simulink model "groudstation20180903"  (R2017b)
settings: Solver=VariableStepAuto  StartTime=0.0  StopTime=inf  RelTol=1e-3
undefined symbols (not defined in the file or in its folder): serial
libraries: instrumentlib x2
settings Model: Creator=E6320  LastModifiedBy=E6320

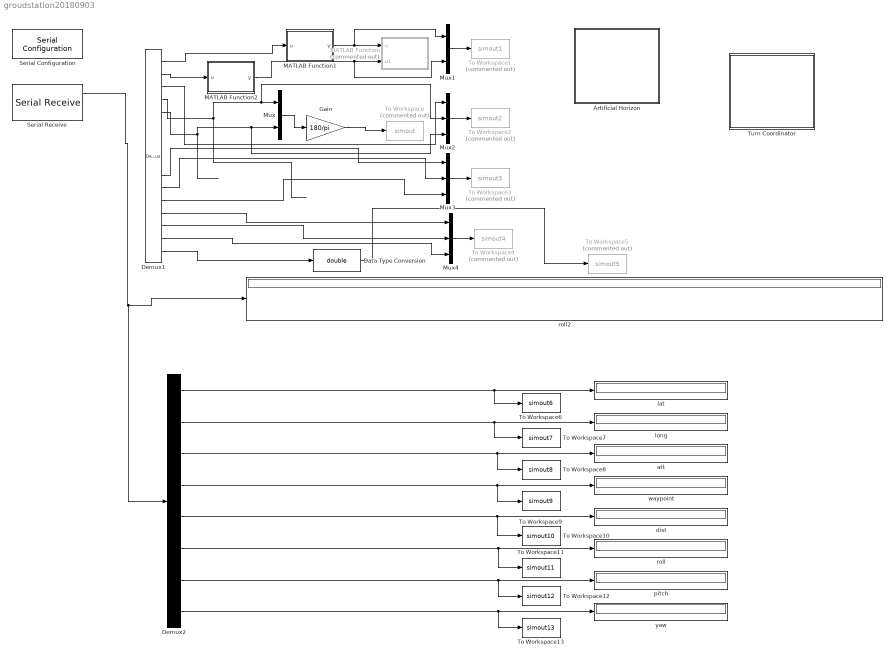
== system groudstation20180903 ==
  Artificial Horizon : Subsystem  DialogController=aeroblksHMICreateDDGDialog  IsWebBlock=on  mask(MWDashboardBlock){webBlockId=80550a31-62cb-4c9e-a581-133f57fb5164, webBlockType=artificialhorizon, ShowInLibBrowser=on, ShowInitialText=on, HMISrcModelName=groudstation20180903}
      mask prompts: webBlockId "WebBlock Id"; webBlockType "WebBlock Type"; HMISrcModelName "Source Model"
      mask help: aeroblksHMI:aeroblkhmi:ArtificialHorizonDialogDesc
      mask Help: eval('asbhmihelp(''artificialhorizon'')');
      mask Display:
      | if strcmp(get_param(bdroot(gcb),'BlockDiagramType'), 'library')
      |  image([(matlabroot) '/toolbox/aeroblks/aeroblks/hmi/icons/ArtificialHorizonIcon.svg'])
      | end
  Data Type Conversion : DataTypeConversion  OutDataTypeStr=double
  Demux1 : Demux  Outputs=16
  Demux2 : Demux  Outputs=8
  Gain : Gain  Gain=180/pi
  MATLAB Function : MATLAB Function  Commented=on  TreatAsAtomicUnit=on
  MATLAB Function1 : MATLAB Function  TreatAsAtomicUnit=on
  MATLAB Function2 : MATLAB Function  TreatAsAtomicUnit=on
  Mux : Mux  Inputs=2
  Mux1 : Mux  Inputs=2
  Mux2 : Mux  Inputs=3
  Mux3 : Mux  Inputs=3
  Mux4 : Mux  Inputs=3
  Serial Configuration : instrumentlib/Serial Configuration  Priority=-200000  ComPortMenu=<Please select a port...>  ComPort=COM12  ObjConstructor=serial('COM12');  BaudRate=57600  DataBits=8  Parity=none  StopBits=1  FlowControl=none  Timeout=10  ByteOrder=LittleEndian
  Serial Receive : instrumentlib/Serial Receive  ComPortMenu=COM12  ComPort=COM12  ObjConstructor=serial('COM12');  Terminator=<none>  DataSize="[8  1]"  DataType=single  EnableBlockingMode=off  ActionDataUnavailable=Output last received value  CustomValue=1  SampleTime=0.5
  To Workspace : ToWorkspace  Commented=on  VariableName=simout  SaveFormat=Timeseries  SampleTime=-1
  To Workspace1 : ToWorkspace  Commented=on  VariableName=simout1  SaveFormat=Timeseries  SampleTime=-1
  To Workspace10 : ToWorkspace  VariableName=simout10  SaveFormat=Timeseries  SampleTime=-1
  To Workspace11 : ToWorkspace  VariableName=simout11  SaveFormat=Timeseries  SampleTime=-1
  To Workspace12 : ToWorkspace  VariableName=simout12  SaveFormat=Timeseries  SampleTime=-1
  To Workspace13 : ToWorkspace  VariableName=simout13  SaveFormat=Timeseries  SampleTime=-1
  To Workspace2 : ToWorkspace  Commented=on  VariableName=simout2  SaveFormat=Timeseries  SampleTime=-1
  To Workspace3 : ToWorkspace  Commented=on  VariableName=simout3  SaveFormat=Timeseries  SampleTime=-1
  To Workspace4 : ToWorkspace  Commented=on  VariableName=simout4  SaveFormat=Timeseries  SampleTime=-1
  To Workspace5 : ToWorkspace  Commented=on  VariableName=simout5  SaveFormat=Timeseries  SampleTime=-1
  To Workspace6 : ToWorkspace  VariableName=simout6  SaveFormat=Timeseries  SampleTime=-1
  To Workspace7 : ToWorkspace  VariableName=simout7  SaveFormat=Timeseries  SampleTime=-1
  To Workspace8 : ToWorkspace  VariableName=simout8  SaveFormat=Timeseries  SampleTime=-1
  To Workspace9 : ToWorkspace  VariableName=simout9  SaveFormat=Timeseries  SampleTime=-1
  Turn Coordinator : Subsystem  DialogController=aeroblksHMICreateDDGDialog  IsWebBlock=on  mask(MWDashboardBlock){webBlockId=99b0b7e4-4174-4c4a-a18a-f9a096f99d10, webBlockType=turncoordinator, ShowInLibBrowser=on, ShowInitialText=on, HMISrcModelName=groudstation20180903}
      mask prompts: webBlockId "WebBlock Id"; webBlockType "WebBlock Type"; HMISrcModelName "Source Model"
      mask help: aeroblksHMI:aeroblkhmi:TurnCoordinatorDialogDesc
      mask Help: eval('asbhmihelp(''turncoordinator'')');
      mask Display:
      | if strcmp(get_param(bdroot(gcb),'BlockDiagramType'), 'library')
      |  image([(matlabroot) '/toolbox/aeroblks/aeroblks/hmi/icons/TurnCoordinatorIcon.svg'])
      | end
  att : Display
  dist : Display
  lat : Display
  long : Display
  pitch : Display
  roll : Display
  roll2 : Display
  waypoint : Display
  yaw : Display
  wires:
  Serial Receive/1 -> Demux2/1, roll2/1
  Mux/1 -> Gain/1
  Gain/1 -> To Workspace/1
  Demux1/4 -> Mux2/2, Mux/1
  Demux1/5 -> Mux2/3, Mux/2
  Demux1/1 -> MATLAB Function1/1(u)
  Demux1/2 -> MATLAB Function2/1(u)
  MATLAB Function1/1(y) -> Mux1/1, MATLAB Function/1(u)
  MATLAB Function2/1(y) -> Mux1/2, MATLAB Function/2(u1)
  Mux1/1 -> To Workspace1/1
  Mux2/1 -> To Workspace2/1
  Demux1/3 -> Mux2/1
  Mux3/1 -> To Workspace3/1
  Demux1/12 -> Mux3/3
  Demux1/11 -> Mux3/2
  Demux1/10 -> Mux3/1
  Mux4/1 -> To Workspace4/1
  Demux1/13 -> Mux4/1
  Demux1/14 -> Mux4/2
  Demux1/15 -> Mux4/3
  Demux1/16 -> Data Type Conversion/1
  Data Type Conversion/1 -> To Workspace5/1
  Demux2/5 -> To Workspace10/1, dist/1
  Demux2/7 -> To Workspace12/1, pitch/1
  Demux2/1 -> To Workspace6/1, lat/1
  Demux2/2 -> To Workspace7/1, long/1
  Demux2/3 -> To Workspace8/1, att/1
  Demux2/4 -> To Workspace9/1, waypoint/1
  Demux2/6 -> To Workspace11/1, roll/1
  Demux2/8 -> To Workspace13/1, yaw/1

== system groudstation20180903/Artificial Horizon ==

== system groudstation20180903/Turn Coordinator ==

== matlab function groudstation20180903/MATLAB Function1 ==
  data: u input; y output
function y = fcn(u)

y = round(u/1000);

== matlab function groudstation20180903/MATLAB Function ==
  data: u input; u1 input
function  fcn(u,u1)
hold on
plot(252000,1214225,'r:diamond')
plot(252007,1214211,'r:diamond')
plot(251985,1214194,'r:diamond')
plot(251979,1214211,'r:diamond')
plot(u,u1,'k:diamond')
end

== matlab function groudstation20180903/MATLAB Function2 ==
  data: u input; y output
function y = fcn(u)

y = round(u/1000);
